simulink model "fifteenlevelconverter"  (R2018a)
settings: Solver=ode45  StartTime=0.0  StopTime=4/50  RelTol=1e-3  EnableMultiTasking=on
InitFcn:
  | fr =60;
  | fc = 22*fr;
  | m = 0.9;
StopFcn:
  | clc
  | 
  | 
  | 
  | 
  | data=power_fftscope(Vab3L)
  | % this portion removes the fundamental and the DC component from the array
  |     temp1=[find(data.freq==0) find(data.freq==60)];
  |     freqf=data.freq;
  |     freqf(temp1)=[];
  |     magf=data.mag;
  |     magf(temp1)=[];
  | % Now calculate the WTHD
  |     WTHD=100*(sqrt(sum((magf./(freqf/data.fundamental)).^2))/data.magFundamental)
  | 
  | 
  | 
  | 
  | data=power_fftscope(VaPD)
  | % this portion removes the fundamental and the DC component from the array
  |     temp1=[find(data.freq==0) find(data.freq==60)];
  |     freqf=data.freq;
  |     freqf(temp1)=[];
  |     magf=data.mag;
  |     magf(temp1)=[];
  | % Now calculate the WTHD
  |     WTHDphase=100*(sqrt(sum((magf./(freqf/data.fundamental)).^2))/data.magFundamental)
libraries: powerlib x16, simulink x14
settings Model: Creator=Luciano Alves  LastModifiedBy=ADHI
settings DataIOCC: LimitDataPoints=on  SaveFormat=Array
settings OptimizationCC: LifeSpan=inf
settings DebuggingCC: UnderspecifiedInitializationDetection=Classic  MergeDetectMultiDrivingBlocksExec=none  SolverPrmCheckMsg=warning  StateNameClashWarn=warning  SFUnexpectedBacktrackingDiag=warning  SFNoUnconditionalDefaultTransitionDiag=warning  SFExecutionAtInitializationDiag=none
settings HardwareCC: ProdBitPerPointer=32  ProdBitPerSizeT=32  ProdBitPerPtrDiffT=32  ProdLargestAtomicFloat=None  ProdIntDivRoundTo=Undefined  ProdEndianess=Unspecified  ProdWordSize=32  ProdHWDeviceType=32-bit Generic
settings ModelReferenceCC: PropagateSignalLabelsOutOfModel=off
settings CodeAppCC: StateflowObjectComments=on
settings GRTTargetCC: TargetLangStandard=C89/C90 (ANSI)  GeneratePreprocessorConditionals=Disable all
settings ConfigComp: CovMetricSettings=dw  CovHtmlReporting=on  CovSaveCumulativeToWorkspaceVar=on  CovSaveSingleToWorkspaceVar=on  CovExternalEMLEnable=off
settings SimscapeCC: SimscapeNormalizeSystem=off

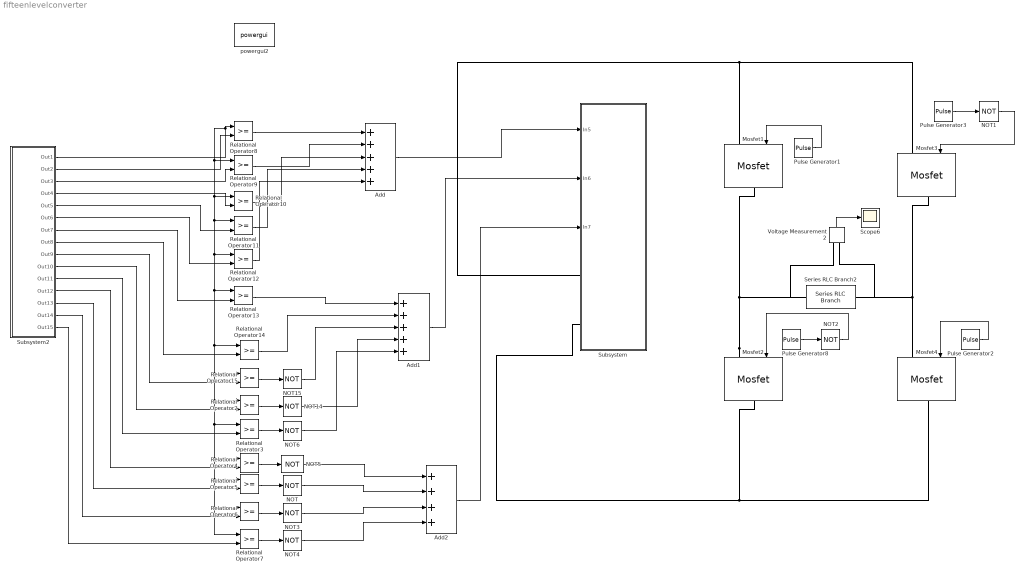
== system fifteenlevelconverter ==
  Add : Sum  Inputs=+++++
  Add1 : Sum  Inputs=+++++
  Add2 : Sum  Inputs=++++
  Mosfet{1..4} (4 alike) : powerlib/Power Electronics/Mosfet  Ron=0.1  Lon=0  Rd=0.01  Vfd=0  IC=0  Rs=1e5  Cs=inf  Measurements=off
  NOT{,1..6,14..15} (9 alike) : Logic  Operator=NOT  IconShape=distinctive  AllPortsSameDT=off  OutDataTypeStr=boolean
  Pulse Generator{1..3,8} (4 alike) : DiscretePulseGenerator  PulseType=Time based  Period=0.02  PulseWidth=50
  Relational Operator{2..15} (14 alike) : RelationalOperator  OutDataTypeStr=boolean  RndMeth=Simplest
  Scope6 : Scope
  Series RLC Branch2 : powerlib/Elements/Series RLC Branch  LConnTagsString=__new0  RConnTagsString=__new0  BranchType=RL  Resistance=420  Inductance=20e-3  SetiL0=off  InitialCurrent=0  Capacitance=1e-6  Setx0=off  InitialVoltage=0  Measurements=None
  Subsystem : Subsystem
  Subsystem2 : Subsystem
  Voltage Measurement2 : powerlib/Measurements/Voltage Measurement  PhasorSimulation=off  OutputType=Complex  PSBequivalent=0
  powergui2 : powerlib/powergui  Priority=1  SimulationMode=Discrete  SampleTime=5e-6  frequency=60  Iterations=50  frequencyindice=0  Pbase=100e6  ErrMax=1e-4  UnitsV=kV  UnitsW=MW  buscounter=0  FunctionMessages=off  echomessages=off  EnableUseOfTLC=off  CurrentSourceSwitches=off  DisableSnubberDevices=off  DisableRonSwitches=off  DisableVfSwitches=off  DisplayEquations=off  SolverType=Tustin  Interpol=off  ExternalGateDelay=off  methode=off  Ts=0  x0status=blocks  SPID=off  SwTol=0  HookPort=off  RestoreLinks=warning  ResistiveCurrentMeasurement=off  Frange=[0:2:500]  Ylog=off  Xlog=on  ShowGrid=off  save=off  variable=ZData  structure=Vlinhapd  ZoomFFT=off  StartTime=0.0  cycles=1  DisplayStyle=1  fundamental=50  FreqAxis=off  MaxFrequency=10000  frequencyindicesteady=1  RmsSteady=1  display=off
  wires:
  Relational Operator15/1 -> NOT15/1
  Pulse Generator8/1 -> NOT2/1
  Pulse Generator1/1 -> Mosfet1/1
  Voltage Measurement2/1 -> Scope6/1
  Pulse Generator3/1 -> NOT1/1
  Pulse Generator2/1 -> Mosfet4/1
  NOT2/1 -> Mosfet2/1
  Relational Operator7/1 -> NOT4/1
  NOT1/1 -> Mosfet3/1
  Relational Operator2/1 -> NOT14/1
  Relational Operator3/1 -> NOT6/1
  Relational Operator4/1 -> NOT5/1
  Relational Operator5/1 -> NOT/1
  Relational Operator6/1 -> NOT3/1
  Subsystem2/1(Out1) -> Relational Operator8/1, Relational Operator7/1, Relational Operator6/1, Relational Operator5/1, Relational Operator4/1, Relational Operator3/1, Relational Operator2/1, Relational Operator15/1, Relational Operator14/1, Relational Operator13/1, Relational Operator12/1, Relational Operator11/1, Relational Operator10/1, Relational Operator9/1
  Subsystem2/2(Out2) -> Relational Operator8/2
  Subsystem2/3(Out3) -> Relational Operator9/2
  Subsystem2/4(Out4) -> Relational Operator10/2
  Subsystem2/5(Out5) -> Relational Operator11/2
  Subsystem2/6(Out6) -> Relational Operator12/2
  Subsystem2/7(Out7) -> Relational Operator13/2
  Subsystem2/8(Out8) -> Relational Operator14/2
  Subsystem2/9(Out9) -> Relational Operator15/2
  Subsystem2/10(Out10) -> Relational Operator2/2
  Subsystem2/11(Out11) -> Relational Operator3/2
  Subsystem2/12(Out12) -> Relational Operator4/2
  Subsystem2/13(Out13) -> Relational Operator5/2
  Subsystem2/14(Out14) -> Relational Operator6/2
  Subsystem2/15(Out15) -> Relational Operator7/2
  Relational Operator8/1 -> Add/1
  Relational Operator9/1 -> Add/2
  Relational Operator10/1 -> Add/3
  Relational Operator11/1 -> Add/4
  Relational Operator12/1 -> Add/5
  Relational Operator13/1 -> Add1/1
  Relational Operator14/1 -> Add1/2
  NOT15/1 -> Add1/3
  NOT14/1 -> Add1/4
  NOT6/1 -> Add1/5
  NOT5/1 -> Add2/1
  NOT/1 -> Add2/2
  NOT3/1 -> Add2/3
  NOT4/1 -> Add2/4
  Add/1 -> Subsystem/1(In5)
  Add1/1 -> Subsystem/2(In6)
  Add2/1 -> Subsystem/3(In7)
  connections:
  Mosfet2/LConn1 -- Voltage Measurement2/LConn1 -- Series RLC Branch2/LConn1 -- Mosfet1/RConn1
  Mosfet3/RConn1 -- Voltage Measurement2/LConn2 -- Series RLC Branch2/RConn1 -- Mosfet4/LConn1
  Mosfet1/LConn1 -- Subsystem/LConn1 -- Mosfet3/LConn1
  Mosfet2/RConn1 -- Subsystem/LConn2 -- Mosfet4/RConn1

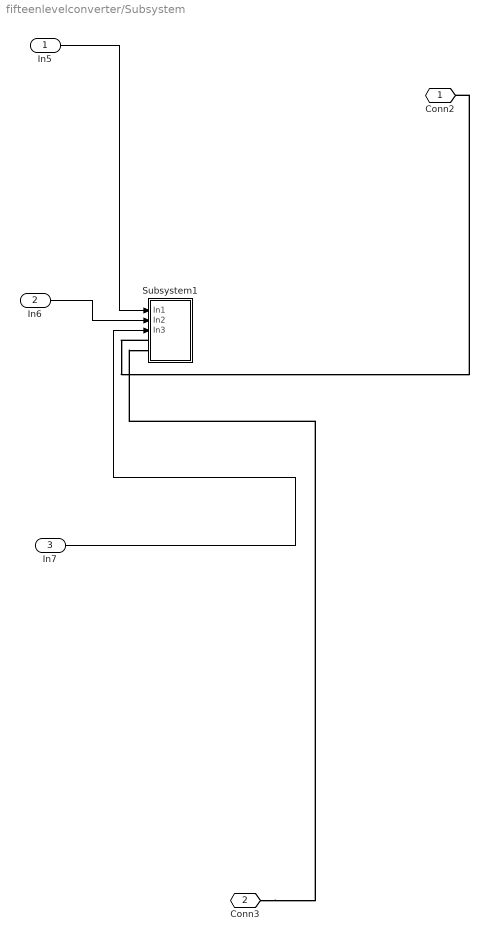
== system fifteenlevelconverter/Subsystem ==
  In5 : Inport
  In6 : Inport  Port=2
  In7 : Inport  Port=3
  Subsystem1 : Subsystem
  Conn2 : PMIOPort  Side=Left
  Conn3 : PMIOPort  Port=2  Side=Left
  wires:
  In6/1 -> Subsystem1/2(In2)
  In7/1 -> Subsystem1/3(In3)
  In5/1 -> Subsystem1/1(In1)
  connections:
  Conn3/RConn1 -- Subsystem1/LConn2
  Subsystem1/LConn1 -- Conn2/RConn1

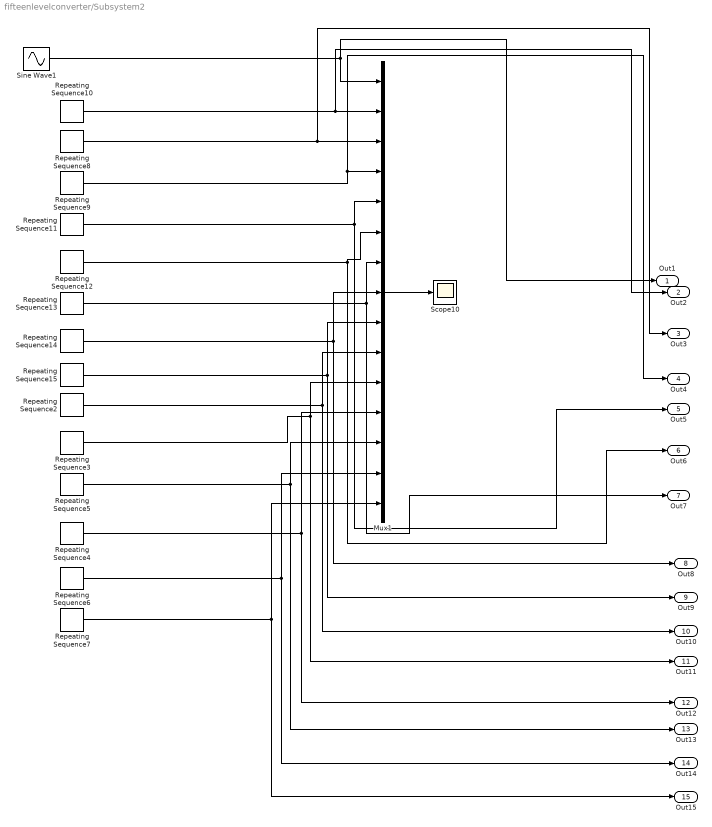
== system fifteenlevelconverter/Subsystem2 ==
  Mux1 : Mux  Inputs=15
  Repeating Sequence10 : simulink/Sources/Repeating Sequence  rep_seq_t=[0 0.00025 0.0005]  rep_seq_y=[6 7 6]
  Repeating Sequence11 : simulink/Sources/Repeating Sequence  rep_seq_t=[0 0.00025 0.0005]  rep_seq_y=[3 4 3]
  Repeating Sequence12 : simulink/Sources/Repeating Sequence  rep_seq_t=[0 0.00025 0.0005]  rep_seq_y=[2 3 2]
  Repeating Sequence13 : simulink/Sources/Repeating Sequence  rep_seq_t=[0 0.00025 0.0005]  rep_seq_y=[1 2 1]
  Repeating Sequence14 : simulink/Sources/Repeating Sequence  rep_seq_t=[0 0.00025 0.0005]  rep_seq_y=[0 1 0]
  Repeating Sequence15 : simulink/Sources/Repeating Sequence  rep_seq_t=[0 0.00025 0.0005]  rep_seq_y=[-1 0 -1]
  Repeating Sequence2 : simulink/Sources/Repeating Sequence  rep_seq_t=[0 0.00025 0.0005]  rep_seq_y=[-2 -1 -2]
  Repeating Sequence3 : simulink/Sources/Repeating Sequence  rep_seq_t=[0 0.00025 0.0005]  rep_seq_y=[-3 -2 -3]
  Repeating Sequence4 : simulink/Sources/Repeating Sequence  rep_seq_t=[0 0.00025 0.0005]  rep_seq_y=[-4 -3 -4]
  Repeating Sequence5 : simulink/Sources/Repeating Sequence  rep_seq_t=[0 0.00025 0.0005]  rep_seq_y=[-5 -4 -5]
  Repeating Sequence6 : simulink/Sources/Repeating Sequence  rep_seq_t=[0 0.00025 0.0005]  rep_seq_y=[-6 -5 -6]
  Repeating Sequence7 : simulink/Sources/Repeating Sequence  rep_seq_t=[0 0.00025 0.0005]  rep_seq_y=[-7 -6 -7]
  Repeating Sequence8 : simulink/Sources/Repeating Sequence  rep_seq_t=[0 0.00025 0.0005]  rep_seq_y=[5 6 5]
  Repeating Sequence9 : simulink/Sources/Repeating Sequence  rep_seq_t=[0 0.00025 0.0005]  rep_seq_y=[4 5 4]
  Scope10 : Scope
  Sine Wave1 : Sin  Amplitude=7  Frequency=2*pi*50  SampleTime=0
  Out1 : Outport
  Out2 : Outport  Port=2
  Out3 : Outport  Port=3
  Out4 : Outport  Port=4
  Out5 : Outport  Port=5
  Out6 : Outport  Port=6
  Out7 : Outport  Port=7
  Out8 : Outport  Port=8
  Out9 : Outport  Port=9
  Out10 : Outport  Port=10
  Out11 : Outport  Port=11
  Out12 : Outport  Port=12
  Out13 : Outport  Port=13
  Out14 : Outport  Port=14
  Out15 : Outport  Port=15
  wires:
  Repeating Sequence13/1 -> Out7/1, Mux1/7
  Repeating Sequence9/1 -> Out4/1, Mux1/4
  Repeating Sequence6/1 -> Out14/1, Mux1/14
  Repeating Sequence12/1 -> Out6/1, Mux1/6
  Sine Wave1/1 -> Out1/1, Mux1/1
  Repeating Sequence15/1 -> Out9/1, Mux1/9
  Repeating Sequence8/1 -> Out3/1, Mux1/3
  Repeating Sequence5/1 -> Out13/1, Mux1/13
  Repeating Sequence7/1 -> Out15/1, Mux1/15
  Repeating Sequence11/1 -> Out5/1, Mux1/5
  Repeating Sequence3/1 -> Out11/1, Mux1/11
  Repeating Sequence2/1 -> Out10/1, Mux1/10
  Repeating Sequence4/1 -> Out12/1, Mux1/12
  Mux1/1 -> Scope10/1
  Repeating Sequence14/1 -> Out8/1, Mux1/8
  Repeating Sequence10/1 -> Out2/1, Mux1/2

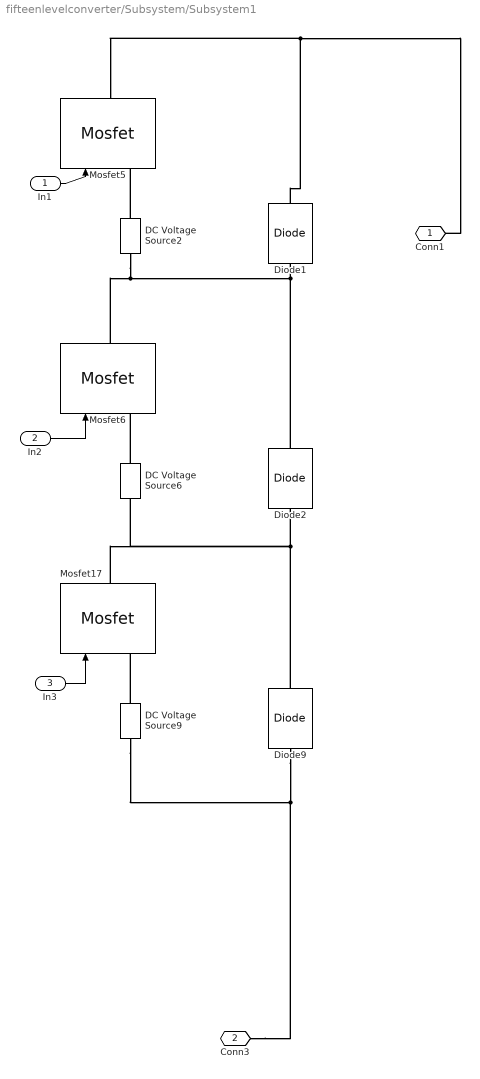
== system fifteenlevelconverter/Subsystem/Subsystem1 ==
  In1 : Inport
  In2 : Inport  Port=2
  In3 : Inport  Port=3
  DC Voltage Source2 : powerlib/Electrical Sources/DC Voltage Source  Amplitude=3  Measurements=None
  DC Voltage Source6 : powerlib/Electrical Sources/DC Voltage Source  Amplitude=6  Measurements=None
  DC Voltage Source9 : powerlib/Electrical Sources/DC Voltage Source  Amplitude=12  Measurements=None
  Diode1 : powerlib/Power Electronics/Diode  Ron=0.001  Lon=0  Vf=0.8  IC=0  UseSnubber=0  Rs=500  Cs=250e-9  Measurements=off
  Diode2 : powerlib/Power Electronics/Diode  Ron=0.001  Lon=0  Vf=0.8  IC=0  UseSnubber=0  Rs=500  Cs=250e-9  Measurements=off
  Diode9 : powerlib/Power Electronics/Diode  Ron=0.001  Lon=0  Vf=0.8  IC=0  UseSnubber=0  Rs=500  Cs=250e-9  Measurements=off
  Mosfet17 : powerlib/Power Electronics/Mosfet  Ron=0.1  Lon=0  Rd=0.01  Vfd=0  IC=0  Rs=1e5  Cs=inf  Measurements=off
  Mosfet5 : powerlib/Power Electronics/Mosfet  Ron=0.1  Lon=0  Rd=0.01  Vfd=0  IC=0  Rs=1e5  Cs=inf  Measurements=off
  Mosfet6 : powerlib/Power Electronics/Mosfet  Ron=0.1  Lon=0  Rd=0.01  Vfd=0  IC=0  Rs=1e5  Cs=inf  Measurements=off
  Conn1 : PMIOPort  Side=Left
  Conn3 : PMIOPort  Port=2  Side=Left
  wires:
  In3/1 -> Mosfet17/1
  In1/1 -> Mosfet5/1
  In2/1 -> Mosfet6/1
  connections:
  DC Voltage Source9/LConn1 -- Diode9/LConn1 -- Conn3/RConn1
  Diode1/RConn1 -- Mosfet5/RConn1 -- Conn1/RConn1
  Diode9/RConn1 -- Mosfet17/RConn1 -- DC Voltage Source6/LConn1 -- Diode2/LConn1
  DC Voltage Source9/RConn1 -- Mosfet17/LConn1
  DC Voltage Source6/RConn1 -- Mosfet6/LConn1
  Mosfet6/RConn1 -- Diode1/LConn1 -- Diode2/RConn1 -- DC Voltage Source2/LConn1
  DC Voltage Source2/RConn1 -- Mosfet5/LConn1
